simulink model "ZVR_Finale"  (R2019b)
settings: Solver=ode23  StartTime=0.0  StopTime=1  MaxStep=1e-5  RelTol=1e-3
libraries: powerlib x23, powerlib_meascontrol x14, dsparch4 x9, simulink x2
settings Model: Creator=ASUS  LastModifiedBy=ASUS
settings SolverCC: ZeroCrossAlgorithm=Adaptive
settings DebuggingCC: IgnoredZcDiagnostic=none

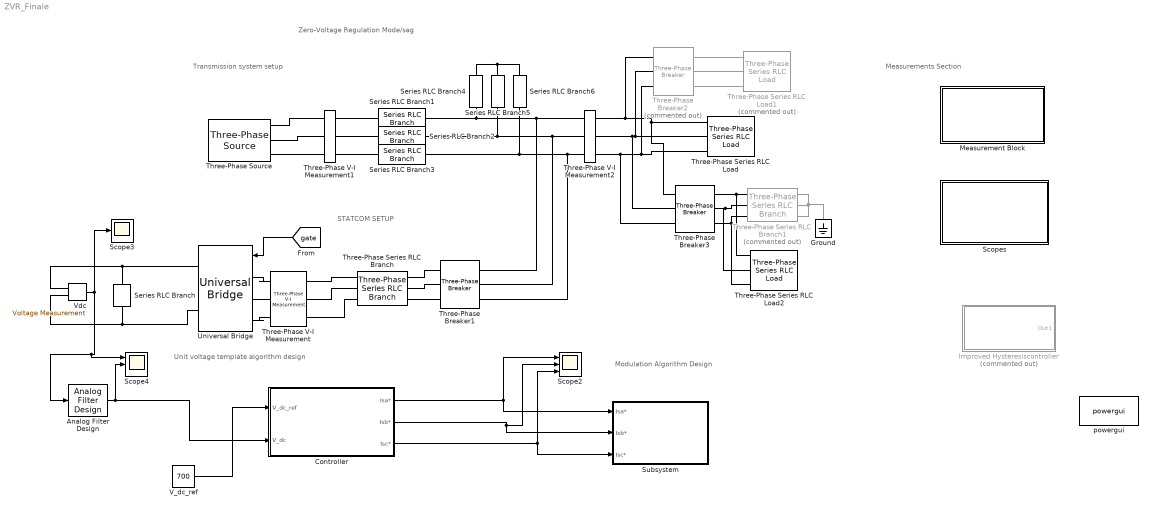
== system ZVR_Finale ==
  note: Zero-Voltage Regulation Mode/sag
  note: Modulation Algorithm Design
  note: Measurements Section
  note: Transmission system setup
  note: Unit voltage template algorithm design
  note: STATCOM SETUP
  Analog Filter Design : dsparch4/Analog Filter Design  method=Butterworth  filttype=Lowpass  N=2  Wlo=100*pi  Whi=80  Rp=2  Rs=40
  Controller : Subsystem
  Ground : powerlib/Elements/Ground  LConnTagsString=a
      settings: SourceProductName=Simscape Electrical
  Improved Hysteresiscontroller : Subsystem  Commented=on
  Measurement Block : Subsystem
  Scope2 : Scope  NumInputPorts=3
  Scope3 : Scope
  Scope4 : Scope  NumInputPorts=3
  Scopes : Subsystem
  Series RLC Branch : powerlib/Elements/Series RLC Branch  LConnTagsString=__new0  RConnTagsString=__new0  BranchType=C  Resistance=1  Inductance=1e-3  SetiL0=off  InitialCurrent=0  Capacitance=10000e-6  Setx0=on  InitialVoltage=700  Measurements=None
      settings: SourceProductName=Simscape Electrical
  Series RLC Branch1 : powerlib/Elements/Series RLC Branch  LConnTagsString=__new0  RConnTagsString=__new0  BranchType=RL  Resistance=0.01  Inductance=1e-3  SetiL0=off  InitialCurrent=0  Capacitance=1e-6  Setx0=off  InitialVoltage=0  Measurements=None
      settings: SourceProductName=Simscape Electrical
  Series RLC Branch2 : powerlib/Elements/Series RLC Branch  LConnTagsString=__new0  RConnTagsString=__new0  BranchType=RL  Resistance=0.01  Inductance=1e-3  SetiL0=off  InitialCurrent=0  Capacitance=1e-6  Setx0=off  InitialVoltage=0  Measurements=None
      settings: SourceProductName=Simscape Electrical
  Series RLC Branch3 : powerlib/Elements/Series RLC Branch  LConnTagsString=__new0  RConnTagsString=__new0  BranchType=RL  Resistance=0.01  Inductance=1e-3  SetiL0=off  InitialCurrent=0  Capacitance=1e-6  Setx0=off  InitialVoltage=0  Measurements=None
      settings: SourceProductName=Simscape Electrical
  Series RLC Branch4 : powerlib/Elements/Series RLC Branch  LConnTagsString=__new0  RConnTagsString=__new0  BranchType=RC  Resistance=5  Inductance=1e-3  SetiL0=off  InitialCurrent=0  Capacitance=5e-6  Setx0=off  InitialVoltage=0  Measurements=None
      settings: SourceProductName=Simscape Electrical
  Series RLC Branch5 : powerlib/Elements/Series RLC Branch  LConnTagsString=__new0  RConnTagsString=__new0  BranchType=RC  Resistance=5  Inductance=1e-3  SetiL0=off  InitialCurrent=0  Capacitance=5e-6  Setx0=off  InitialVoltage=0  Measurements=None
      settings: SourceProductName=Simscape Electrical
  Series RLC Branch6 : powerlib/Elements/Series RLC Branch  LConnTagsString=__new0  RConnTagsString=__new0  BranchType=RC  Resistance=5  Inductance=1e-3  SetiL0=off  InitialCurrent=0  Capacitance=5e-6  Setx0=off  InitialVoltage=0  Measurements=None
      settings: SourceProductName=Simscape Electrical
  Subsystem : Subsystem
  Three-Phase Series RLC Branch : powerlib/Elements/Three-Phase Series RLC Branch  LConnTagsString=A|B|C  RConnTagsString=A|B|C  BranchType=RL  Resistance=0.1  Inductance=4e-3  Capacitance=0  Measurements=None
      settings: SourceProductName=Simscape Electrical
  Three-Phase Series RLC Branch1 : powerlib/Elements/Three-Phase Series RLC Branch  Commented=on  LConnTagsString=A|B|C  RConnTagsString=A|B|C  BranchType=RL  Resistance=0.01  Inductance=10e-3  Capacitance=1e-6  Measurements=None
      settings: SourceProductName=Simscape Electrical
  Three-Phase Series RLC Load : powerlib/Elements/Three-Phase Series RLC Load  LConnTagsString=A|B|C  Configuration=Y (grounded)  NominalVoltage=415  Vabc=[1e3 1e3 1e3]  Vabcp=[1e3 1e3 1e3]  NominalFrequency=50  UnbalancedPower=off  ActivePower=3000  InductivePower=7000  CapacitivePower=0  Pabc=[10e3 9e3 11e3]  QLabc=[100 90 110]  QCabc=[100 90 110]  Pabcp=[10e3 9e3 11e3]  QLabcp=[100 90 110]  QCabcp=[100 90 110]  Measurements=None  LoadType=constant Z
      settings: SourceProductName=Simscape Electrical
  Three-Phase Series RLC Load1 : powerlib/Elements/Three-Phase Series RLC Load  Commented=on  LConnTagsString=A|B|C  Configuration=Y (grounded)  NominalVoltage=415  Vabc=[1e3 1e3 1e3]  Vabcp=[1e3 1e3 1e3]  NominalFrequency=50  UnbalancedPower=off  ActivePower=10e4  InductivePower=3000  CapacitivePower=0  Pabc=[10e3 9e3 11e3]  QLabc=[100 90 110]  QCabc=[100 90 110]  Pabcp=[10e3 9e3 11e3]  QLabcp=[100 90 110]  QCabcp=[100 90 110]  Measurements=None  LoadType=constant Z
      settings: SourceProductName=Simscape Electrical
  Three-Phase Series RLC Load2 : powerlib/Elements/Three-Phase Series RLC Load  LConnTagsString=A|B|C  Configuration=Y (grounded)  NominalVoltage=415  Vabc=[1e3 1e3 1e3]  Vabcp=[1e3 1e3 1e3]  NominalFrequency=50  UnbalancedPower=off  ActivePower=200  InductivePower=10000  CapacitivePower=0  Pabc=[10e3 9e3 11e3]  QLabc=[100 90 110]  QCabc=[100 90 110]  Pabcp=[10e3 9e3 11e3]  QLabcp=[100 90 110]  QCabcp=[100 90 110]  Measurements=None  LoadType=constant Z
      settings: SourceProductName=Simscape Electrical
  Three-Phase V-I Measurement : powerlib/Measurements/Three-Phase V-I Measurement  VoltageMeasurement=phase-to-ground  SetLabelV=on  LabelV=V_stat  Vpu=off  VpuLL=off  CurrentMeasurement=yes  SetLabelI=on  LabelI=I_stat  Ipu=off  Pbase=100e6  Vbase=500e3  OutputType=Complex  PhasorSimulation=off  PSBequivalent=0
      settings: SourceProductName=Simscape Electrical
  Three-Phase V-I Measurement1 : powerlib/Measurements/Three-Phase V-I Measurement  VoltageMeasurement=phase-to-ground  SetLabelV=on  LabelV=Vs  Vpu=off  VpuLL=off  CurrentMeasurement=yes  SetLabelI=on  LabelI=Is  Ipu=off  Pbase=100e6  Vbase=500e3  OutputType=Complex  PhasorSimulation=off  PSBequivalent=0
      settings: SourceProductName=Simscape Electrical
  Three-Phase V-I Measurement2 : powerlib/Measurements/Three-Phase V-I Measurement  VoltageMeasurement=phase-to-ground  SetLabelV=on  LabelV=Vr  Vpu=off  VpuLL=off  CurrentMeasurement=yes  SetLabelI=on  LabelI=Ir  Ipu=off  Pbase=100e6  Vbase=500e3  OutputType=Complex  PhasorSimulation=off  PSBequivalent=0
      settings: SourceProductName=Simscape Electrical
  Three-Phase Breaker1 : powerlib/Elements/Three-Phase Breaker  InitialState=open  SwitchA=on  SwitchB=on  SwitchC=on  SwitchTimes=[0.2 0.6]  External=off  BreakerResistance=0.01  SnubberResistance=1e6  SnubberCapacitance=inf  Measurements=None
      settings: SourceProductName=Simscape Electrical
  Three-Phase Breaker2 : powerlib/Elements/Three-Phase Breaker  Commented=on  InitialState=open  SwitchA=on  SwitchB=on  SwitchC=on  SwitchTimes=[0.1 0.5]  External=off  BreakerResistance=0.01  SnubberResistance=1e6  SnubberCapacitance=inf  Measurements=None
      settings: SourceProductName=Simscape Electrical
  Three-Phase Breaker3 : powerlib/Elements/Three-Phase Breaker  InitialState=open  SwitchA=on  SwitchB=on  SwitchC=on  SwitchTimes=[0.1 0.6]  External=off  BreakerResistance=0.01  SnubberResistance=1e6  SnubberCapacitance=inf  Measurements=None
      settings: SourceProductName=Simscape Electrical
  Three-Phase Source : powerlib/Electrical Sources/Three-Phase Source  InternalConnection=Yg  VoltagePhases=off  Voltage=415  PhaseAngle=0  Voltage_phases=[25e3 25e3 25e3]/sqrt(3)  PhaseAngles_phases=[0 -120 +120]  Frequency=50  NonIdealSource=on  SpecifyImpedance=off  Resistance=0.04  Inductance=0.5e-3  ShortCircuitLevel=100e6  BaseVoltage=415  XRratio=7  BusType=swing  Pref=10e3  Qref=0  Prefabc=[10e3, 10e3, 10e3]  Qrefabc=[0, 0, 0]  Qmin=-inf  Qmax=inf
      settings: SourceProductName=Simscape Electrical
  Universal Bridge : powerlib/Power Electronics/Universal Bridge  Arms=3  SnubberResistance=1e5  SnubberCapacitance=inf  Device=IGBT / Diodes  Ron=1e-3  Lon=0  ForwardVoltages="[  0  0  ]"  ForwardVoltage=0  GTOparameters=[ 10e-6 , 20e-6 ]  IGBTparameters=[ 1e-6 , 2e-6 ]  Measurements=None  Measurements_2=None  converterType=Rectifier
      settings: SourceProductName=Simscape Electrical
  V_dc_ref : Constant  Value=700
  Vdc : powerlib/Measurements/Voltage Measurement  PhasorSimulation=off  OutputType=Complex  PSBequivalent=0
      settings: SourceProductName=Simscape Electrical
  powergui : powerlib/powergui  Priority=1  SimulationMode=Discrete  SampleTime=1e-6  frequency=60  Iterations=50  frequencyindice=0  Pbase=100e6  ErrMax=1e-4  UnitsV=kV  UnitsW=MW  buscounter=0  FunctionMessages=off  echomessages=off  EnableUseOfTLC=off  CurrentSourceSwitches=off  DisableSnubberDevices=off  DisableRonSwitches=off  DisableVfSwitches=off  DisplayEquations=off  AutomaticDiscreteSolvers=off  SolverType=Tustin/Backward Euler (TBE)  Interpol=off  ExternalGateDelay=off  methode=off  Ts=100  x0status=blocks  SPID=on  SwTol=0  HookPort=off  NonlinearTolerance=1e-4  nMaxIteration=100  ContinueOnMaxIteration=off  RestoreLinks=warning  ResistiveCurrentMeasurement=off  Frange=[0:2:500]  Ylog=off  Xlog=on  ShowGrid=off  save=off  variable=ZData  structure=0  ZoomFFT=off  StartTime=0.0  cycles=1  DisplayStyle=1  fundamental=60  FreqAxis=off  MaxFrequency=1000  frequencyindicesteady=1  RmsSteady=1  display=off
      settings: SourceProductName=Simscape Electrical
  wires:
  V_dc_ref/1 -> Controller/1(V_dc_ref)
  Controller/1(Isa*) -> Subsystem/1(Isa*), Scope2/1
  Controller/2(Isb*) -> Subsystem/2(Isb*), Scope2/2
  Controller/3(Isc*) -> Subsystem/3(Isc*), Scope2/3
  Vdc/1 -> Scope4/1, Analog Filter Design/1, Scope3/1
  Analog Filter Design/1 -> Scope4/2, Controller/2(V_dc)
  [gate] -> Universal Bridge/1
  connections:
  Three-Phase Source/RConn1 -- Three-Phase V-I Measurement1/LConn1
  Three-Phase Source/RConn2 -- Three-Phase V-I Measurement1/LConn2
  Three-Phase Source/RConn3 -- Three-Phase V-I Measurement1/LConn3
  Series RLC Branch5/LConn1 -- Series RLC Branch2/RConn1 -- Three-Phase Breaker1/RConn2 -- Three-Phase V-I Measurement2/LConn2
  Series RLC Branch6/LConn1 -- Series RLC Branch3/RConn1 -- Three-Phase Breaker1/RConn3 -- Three-Phase V-I Measurement2/LConn3
  Three-Phase Series RLC Load/LConn1 -- Three-Phase Breaker2/LConn1 -- Three-Phase V-I Measurement2/RConn1 -- Three-Phase Breaker3/LConn1
  Three-Phase Series RLC Load/LConn2 -- Three-Phase Breaker3/LConn2 -- Three-Phase V-I Measurement2/RConn2 -- Three-Phase Breaker2/LConn2
  Three-Phase V-I Measurement2/RConn3 -- Three-Phase Breaker3/LConn3 -- Three-Phase Breaker2/LConn3 -- Three-Phase Series RLC Load/LConn3
  Series RLC Branch4/LConn1 -- Series RLC Branch1/RConn1 -- Three-Phase Breaker1/RConn1 -- Three-Phase V-I Measurement2/LConn1
  Series RLC Branch4/RConn1 -- Series RLC Branch6/RConn1 -- Series RLC Branch5/RConn1
  Series RLC Branch/LConn1 -- Vdc/LConn1 -- Universal Bridge/RConn1
  Series RLC Branch/RConn1 -- Universal Bridge/RConn2 -- Vdc/LConn2
  Three-Phase Series RLC Branch/RConn3 -- Three-Phase Breaker1/LConn3
  Three-Phase Series RLC Branch/RConn1 -- Three-Phase Breaker1/LConn1
  Three-Phase Series RLC Branch/RConn2 -- Three-Phase Breaker1/LConn2
  Three-Phase V-I Measurement/LConn1 -- Universal Bridge/LConn1
  Universal Bridge/LConn2 -- Three-Phase V-I Measurement/LConn2
  Universal Bridge/LConn3 -- Three-Phase V-I Measurement/LConn3
  Three-Phase V-I Measurement/RConn1 -- Three-Phase Series RLC Branch/LConn1
  Three-Phase V-I Measurement/RConn2 -- Three-Phase Series RLC Branch/LConn2
  Three-Phase V-I Measurement/RConn3 -- Three-Phase Series RLC Branch/LConn3
  Series RLC Branch1/LConn1 -- Three-Phase V-I Measurement1/RConn1
  Series RLC Branch2/LConn1 -- Three-Phase V-I Measurement1/RConn2
  Series RLC Branch3/LConn1 -- Three-Phase V-I Measurement1/RConn3
  Three-Phase Breaker2/RConn1 -- Three-Phase Series RLC Load1/LConn1
  Three-Phase Breaker2/RConn2 -- Three-Phase Series RLC Load1/LConn2
  Three-Phase Breaker2/RConn3 -- Three-Phase Series RLC Load1/LConn3
  Three-Phase Series RLC Branch1/RConn1 -- Ground/LConn1 -- Three-Phase Series RLC Branch1/RConn2 -- Three-Phase Series RLC Branch1/RConn3
  Three-Phase Breaker3/RConn1 -- Three-Phase Series RLC Load2/LConn1 -- Three-Phase Series RLC Branch1/LConn1
  Three-Phase Breaker3/RConn2 -- Three-Phase Series RLC Branch1/LConn2 -- Three-Phase Series RLC Load2/LConn2
  Three-Phase Breaker3/RConn3 -- Three-Phase Series RLC Load2/LConn3 -- Three-Phase Series RLC Branch1/LConn3

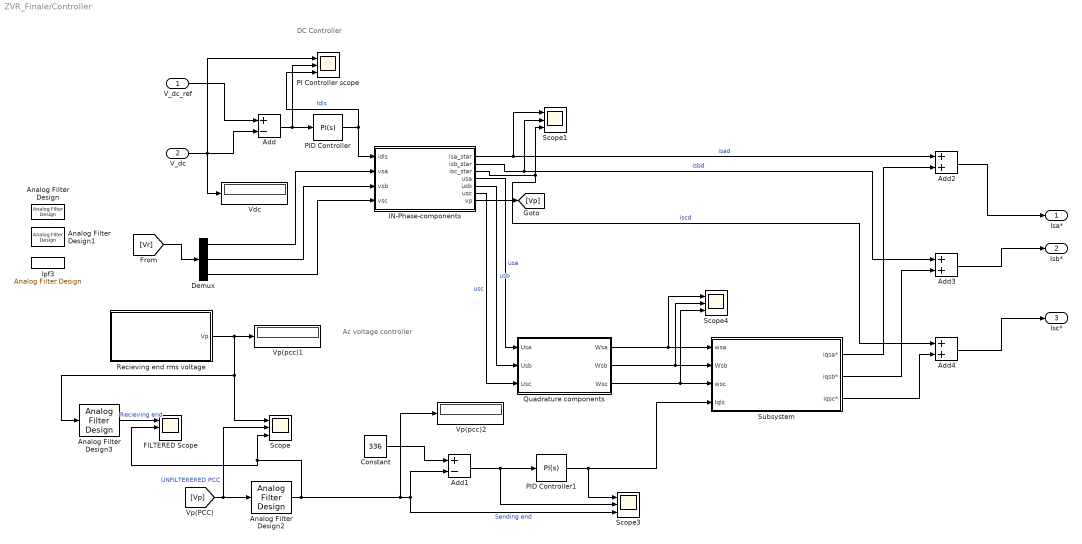
== system ZVR_Finale/Controller ==
  note: Ac voltage controller
  note: DC Controller
  V_dc_ref : Inport
  V_dc : Inport  Port=2
  Add : Sum  Inputs=+-
  Add1 : Sum  Inputs=+-
  Add2 : Sum
  Add3 : Sum
  Add4 : Sum
  Analog Filter Design : dsparch4/Analog Filter Design  method=Butterworth  filttype=Lowpass  N=2  Wlo=20000*2*pi  Whi=80  Rp=2  Rs=40
  Analog Filter Design1 : dsparch4/Analog Filter Design  method=Butterworth  filttype=Lowpass  N=2  Wlo=20000*2*pi  Whi=80  Rp=2  Rs=40
  Analog Filter Design2 : dsparch4/Analog Filter Design  method=Butterworth  filttype=Lowpass  N=2  Wlo=50*pi  Whi=80  Rp=2  Rs=40
  Analog Filter Design3 : dsparch4/Analog Filter Design  method=Butterworth  filttype=Lowpass  N=2  Wlo=50*pi  Whi=80  Rp=2  Rs=40
  Constant : Constant  Value=336
  Demux : Demux  Outputs=3
  FILTERED Scope : Scope  NumInputPorts=3
  IN-Phase-components : MATLAB Function  TreatAsAtomicUnit=on
  PI Controller scope : Scope  NumInputPorts=3
  PID Controller : simulink/Continuous/PID Controller  Controller=PI  Form=Parallel  TimeDomain=Continuous-time  SampleTime=-1  IntegratorMethod=Forward Euler  FilterMethod=Forward Euler  ControllerParametersSource=internal  P=3  I=8  D=0  UseFilter=on  N=100  TunerSelectOption=Transfer Function Based (PID Tuner App)  InitialConditionSource=internal  InitialConditionForIntegrator=0  InitialConditionForFilter=0  DifferentiatorICPrevScaledInput=0  ExternalReset=none  TrackingMode=off  Kt=1  LimitOutput=off  UpperSaturationLimit=inf  LowerSaturationLimit=-inf  LinearizeAsGain=on  AntiWindupMode=none  Kb=1  POutMin=[]  POutMax=[]  IOutMin=[]  IOutMax=[]  DOutMin=[]  DOutMax=[]  NOutMin=[]  NOutMax=[]  SumOutMin=[]  SumOutMax=[]  SaturationOutMin=[]  SaturationOutMax=[]  PParamMin=[]  PParamMax=[]  IParamMin=[]  IParamMax=[]  DParamMin=[]  DParamMax=[]  NParamMin=[]  NParamMax=[]  KbParamMin=[]  KbParamMax=[]  KtParamMin=[]  KtParamMax=[]  KbOutMin=[]  KbOutMax=[]  KtOutMin=[]  KtOutMax=[]  IntegratorOutMin=[]  IntegratorOutMax=[]  FilterOutMin=[]  FilterOutMax=[]  SumI1OutMin=[]  SumI1OutMax=[]  SumI2OutMin=[]  SumI2OutMax=[]  SumI3OutMin=[]  SumI3OutMax=[]  SumI4OutMin=[]  SumI4OutMax=[]  SumDOutMin=[]  SumDOutMax=[]  DifferentiatorOutMin=[]  DifferentiatorOutMax=[]  FilterDiffOutCoefMin=[]  FilterDiffOutCoefMax=[]  ReciprocalOutMin=[]  ReciprocalOutMax=[]  SumDenOutMin=[]  SumDenOutMax=[]  SumNumOutMin=[]  SumNumOutMax=[]  DivideOutMin=[]  DivideOutMax=[]  IntegratorContinuousStateAttributes=''  IntegratorStateMustResolveToSignalObject=off  IntegratorRTWStateStorageClass=Auto  FilterContinuousStateAttributes=''  FilterStateMustResolveToSignalObject=off  FilterRTWStateStorageClass=Auto  ParallelPVariant=InternalParameters  IdealPVariant=Disabled  IVariant=InternalParameters  DVariant=Disabled  IntegratorVariant=Continuous  SatVariant=Disabled  AWVariant=Passthrough  PCopyVariant=Disabled  TRVariant=Disabled  FdbkBlocksVariant=Forward  IdealPFdbkVariant=Disabled  SatFdbkVariant=Disabled  DerivativeFilterVariant=Disabled  NVariant=Disabled  NCopyVariant=Disabled_SignalSpec  FilterICVariant=Disabled  IntegratorICVariant=InternalICs  ExternalResetVariant=Disabled  TRSumVariant=Passthrough  SumFdbkVariant=Disabled  SumVariant=Sum_PI
  PID Controller1 : simulink/Continuous/PID Controller  Controller=PI  Form=Parallel  TimeDomain=Continuous-time  SampleTime=-1  IntegratorMethod=Forward Euler  FilterMethod=Forward Euler  ControllerParametersSource=internal  P=1.2  I=0.6  D=0  UseFilter=on  N=100  TunerSelectOption=Transfer Function Based (PID Tuner App)  InitialConditionSource=internal  InitialConditionForIntegrator=0  InitialConditionForFilter=0  DifferentiatorICPrevScaledInput=0  ExternalReset=none  TrackingMode=off  Kt=1  LimitOutput=off  UpperSaturationLimit=inf  LowerSaturationLimit=-inf  LinearizeAsGain=on  AntiWindupMode=none  Kb=1  POutMin=[]  POutMax=[]  IOutMin=[]  IOutMax=[]  DOutMin=[]  DOutMax=[]  NOutMin=[]  NOutMax=[]  SumOutMin=[]  SumOutMax=[]  SaturationOutMin=[]  SaturationOutMax=[]  PParamMin=[]  PParamMax=[]  IParamMin=[]  IParamMax=[]  DParamMin=[]  DParamMax=[]  NParamMin=[]  NParamMax=[]  KbParamMin=[]  KbParamMax=[]  KtParamMin=[]  KtParamMax=[]  KbOutMin=[]  KbOutMax=[]  KtOutMin=[]  KtOutMax=[]  IntegratorOutMin=[]  IntegratorOutMax=[]  FilterOutMin=[]  FilterOutMax=[]  SumI1OutMin=[]  SumI1OutMax=[]  SumI2OutMin=[]  SumI2OutMax=[]  SumI3OutMin=[]  SumI3OutMax=[]  SumI4OutMin=[]  SumI4OutMax=[]  SumDOutMin=[]  SumDOutMax=[]  DifferentiatorOutMin=[]  DifferentiatorOutMax=[]  FilterDiffOutCoefMin=[]  FilterDiffOutCoefMax=[]  ReciprocalOutMin=[]  ReciprocalOutMax=[]  SumDenOutMin=[]  SumDenOutMax=[]  SumNumOutMin=[]  SumNumOutMax=[]  DivideOutMin=[]  DivideOutMax=[]  IntegratorContinuousStateAttributes=''  IntegratorStateMustResolveToSignalObject=off  IntegratorRTWStateStorageClass=Auto  FilterContinuousStateAttributes=''  FilterStateMustResolveToSignalObject=off  FilterRTWStateStorageClass=Auto  ParallelPVariant=InternalParameters  IdealPVariant=Disabled  IVariant=InternalParameters  DVariant=Disabled  IntegratorVariant=Continuous  SatVariant=Disabled  AWVariant=Passthrough  PCopyVariant=Disabled  TRVariant=Disabled  FdbkBlocksVariant=Forward  IdealPFdbkVariant=Disabled  SatFdbkVariant=Disabled  DerivativeFilterVariant=Disabled  NVariant=Disabled  NCopyVariant=Disabled_SignalSpec  FilterICVariant=Disabled  IntegratorICVariant=InternalICs  ExternalResetVariant=Disabled  TRSumVariant=Passthrough  SumFdbkVariant=Disabled  SumVariant=Sum_PI
  "Quadrature components " : Subsystem
  Recieving end rms voltage : Subsystem
  Scope{,1,3..4} (4 alike) : Scope  NumInputPorts=3
  Subsystem : Subsystem
  Vdc : Display
  Vp(pcc)1 : Display
  Vp(pcc)2 : Display
  lpf3 : dsparch4/Analog Filter Design  method=Butterworth  filttype=Lowpass  N=2  Wlo=20000*2*pi  Whi=80  Rp=2  Rs=40
  Isa* : Outport
  Isb* : Outport  Port=2
  Isc* : Outport  Port=3
  wires:
  V_dc_ref/1 -> Add/1
  V_dc/1 -> PI Controller scope/1, Add/2, Vdc/1
  Add/1 -> PI Controller scope/2, PID Controller/1
  PID Controller/1 -> PI Controller scope/3, IN-Phase-components/1(idls)  "Idls"
  [Vr] -> Demux/1
  IN-Phase-components/1(isa_star) -> Add2/1, Scope1/1  "isad"
  IN-Phase-components/2(isb_star) -> Add3/1, Scope1/2  "isbd"
  IN-Phase-components/3(isc_star) -> Add4/1, Scope1/3  "iscd"
  IN-Phase-components/4(usa) -> "Quadrature components "/1(Usa)  "usa"
  IN-Phase-components/5(usb) -> "Quadrature components "/2(Usb)  "usb"
  IN-Phase-components/6(usc) -> "Quadrature components "/3(Usc)  "usc"
  Demux/1 -> IN-Phase-components/2(vsa)
  Demux/2 -> IN-Phase-components/3(vsb)
  Demux/3 -> IN-Phase-components/4(vsc)
  "Quadrature components "/1(Wsa) -> Scope4/1, Subsystem/1(wsa)
  Recieving end rms voltage/1(Vp) -> Analog Filter Design3/1, Scope/1, Vp(pcc)1/1
  IN-Phase-components/7(vp) -> [Vp]
  Constant/1 -> Add1/1
  Analog Filter Design2/1 -> Scope/3, FILTERED Scope/2, Vp(pcc)2/1, Add1/2, Scope3/3  "Sending end"
  Add1/1 -> Scope3/2, PID Controller1/1
  PID Controller1/1 -> Scope3/1, Subsystem/4(Iqls)
  "Quadrature components "/2(Wsb) -> Scope4/2, Subsystem/2(Wsb)
  "Quadrature components "/3(Wsc) -> Scope4/3, Subsystem/3(wsc)
  Subsystem/1(iqsa*) -> Add2/2
  Add2/1 -> Isa*/1
  Subsystem/2(iqsb*) -> Add3/2
  Subsystem/3(iqsc*) -> Add4/2
  Add3/1 -> Isb*/1
  Add4/1 -> Isc*/1
  [Vp] -> Scope/2, Analog Filter Design2/1  "UNFILTERERED PCC"
  Analog Filter Design3/1 -> FILTERED Scope/1  "Recieving end"

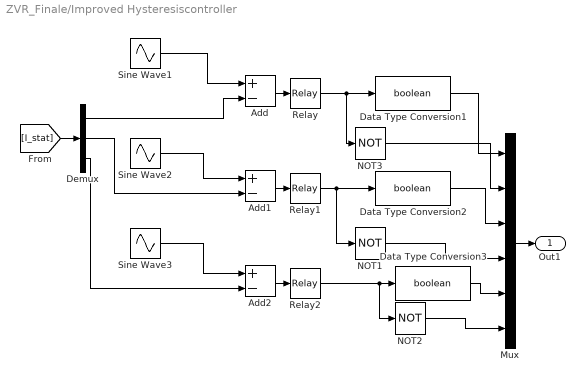
== system ZVR_Finale/Improved Hysteresiscontroller ==
  Add : Sum  Inputs=+-
  Add1 : Sum  Inputs=+-
  Add2 : Sum  Inputs=+-
  Data Type Conversion1 : DataTypeConversion  OutDataTypeStr=boolean
  Data Type Conversion2 : DataTypeConversion  OutDataTypeStr=boolean
  Data Type Conversion3 : DataTypeConversion  OutDataTypeStr=boolean
  Demux : Demux  Outputs=3
  Mux : Mux  Inputs=6
  NOT1 : Logic  Operator=NOT  IconShape=distinctive  AllPortsSameDT=off  OutDataTypeStr=boolean
  NOT2 : Logic  Operator=NOT  IconShape=distinctive  AllPortsSameDT=off  OutDataTypeStr=boolean
  NOT3 : Logic  Operator=NOT  IconShape=distinctive  AllPortsSameDT=off  OutDataTypeStr=boolean
  Relay : Relay  OnSwitchValue=0.1  OffSwitchValue=-0.1
  Relay1 : Relay  OnSwitchValue=0.1  OffSwitchValue=-0.1
  Relay2 : Relay  OnSwitchValue=0.1  OffSwitchValue=-0.1
  Sine Wave1 : Sin  Amplitude=5  Frequency=100*pi  SampleTime=0
  Sine Wave2 : Sin  Amplitude=5  Frequency=100*pi  Phase=-2*pi/3  SampleTime=0
  Sine Wave3 : Sin  Amplitude=5  Frequency=100*pi  Phase=2*pi/3  SampleTime=0
  Out1 : Outport
  wires:
  Data Type Conversion3/1 -> Mux/5
  Relay/1 -> NOT3/1, Data Type Conversion1/1
  Sine Wave1/1 -> Add/1
  Add2/1 -> Relay2/1
  Sine Wave2/1 -> Add1/1
  Relay1/1 -> NOT1/1, Data Type Conversion2/1
  Sine Wave3/1 -> Add2/1
  Data Type Conversion1/1 -> Mux/1
  NOT1/1 -> Mux/4
  NOT3/1 -> Mux/2
  Add1/1 -> Relay1/1
  Relay2/1 -> Data Type Conversion3/1, NOT2/1
  [I_stat] -> Demux/1
  Demux/2 -> Add1/2
  Add/1 -> Relay/1
  Demux/1 -> Add/2
  NOT2/1 -> Mux/6
  Data Type Conversion2/1 -> Mux/3
  Demux/3 -> Add2/2
  Mux/1 -> Out1/1

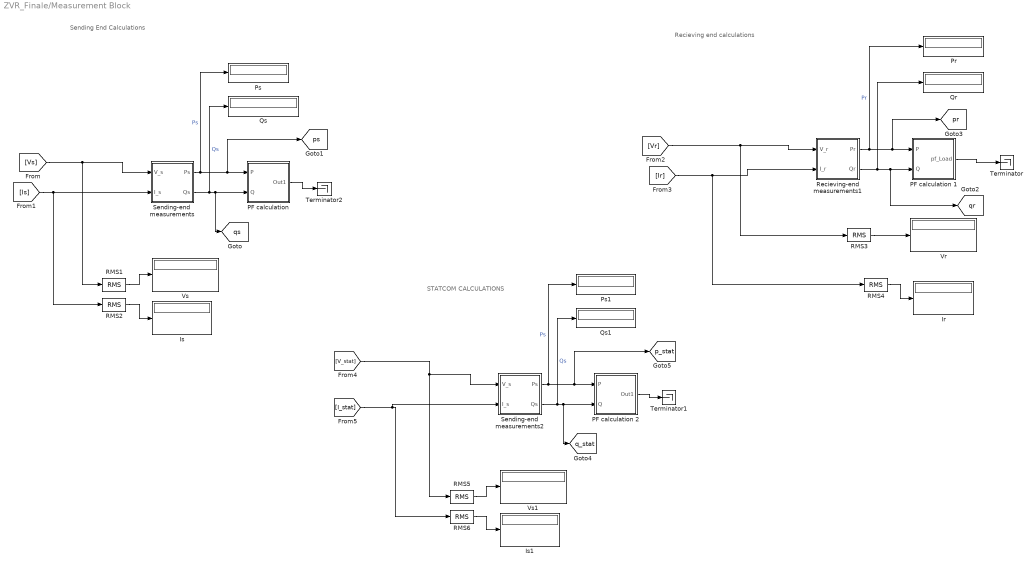
== system ZVR_Finale/Measurement Block ==
  note: STATCOM CALCULATIONS
  note: Recieving end calculations
  note: Sending End Calculations
  Ir : Display
  Is : Display
  Is1 : Display
  "PF calculation " : Subsystem
  PF calculation 1 : Subsystem
  PF calculation 2 : Subsystem
  Pr : Display
  Ps : Display
  Ps1 : Display
  Qr : Display
  Qs : Display
      settings: Format=short_e
  Qs1 : Display
  RMS{1..6} (6 alike) : powerlib_meascontrol/Measurements/RMS  TrueRMS=on  Freq=60  RMSInit=120  Ts=0
      settings: SourceProductName=Simscape Electrical
  Recieving-end measurements1 : Subsystem
  Sending-end measurements : Subsystem
  Sending-end measurements2 : Subsystem
  Terminator : Terminator
  Terminator1 : Terminator
  Terminator2 : Terminator
  Vr : Display
  Vs : Display
  Vs1 : Display
  tag scope: p_stat=global, pr=global, ps=global, q_stat=global, qr=global, qs=global
  wires:
  Sending-end measurements/1(Ps) -> Ps/1, [ps], "PF calculation "/1(P)  "Ps"
  Sending-end measurements/2(Qs) -> Qs/1, [qs], "PF calculation "/2(Q)  "Qs"
  [Is] -> RMS2/1, Sending-end measurements/2(I_s)
  Recieving-end measurements1/2(Qr) -> Qr/1, [qr], PF calculation 1/2(Q)
  Recieving-end measurements1/1(Pr) -> Pr/1, [pr], PF calculation 1/1(P)  "Pr"
  RMS1/1 -> Vs/1
  RMS2/1 -> Is/1
  [Vs] -> Sending-end measurements/1(V_s), RMS1/1
  RMS3/1 -> Vr/1
  [Vr] -> RMS3/1, Recieving-end measurements1/1(V_r)
  RMS4/1 -> Ir/1
  [Ir] -> RMS4/1, Recieving-end measurements1/2(I_r)
  Sending-end measurements2/2(Qs) -> Qs1/1, [q_stat], PF calculation 2/2(Q)  "Qs"
  Sending-end measurements2/1(Ps) -> Ps1/1, [p_stat], PF calculation 2/1(P)  "Ps"
  [V_stat] -> Sending-end measurements2/1(V_s), RMS5/1
  RMS5/1 -> Vs1/1
  RMS6/1 -> Is1/1
  [I_stat] -> Sending-end measurements2/2(I_s), RMS6/1
  PF calculation 1/1(pf_Load) -> Terminator/1
  PF calculation 2/1(Out1) -> Terminator1/1
  "PF calculation "/1(Out1) -> Terminator2/1

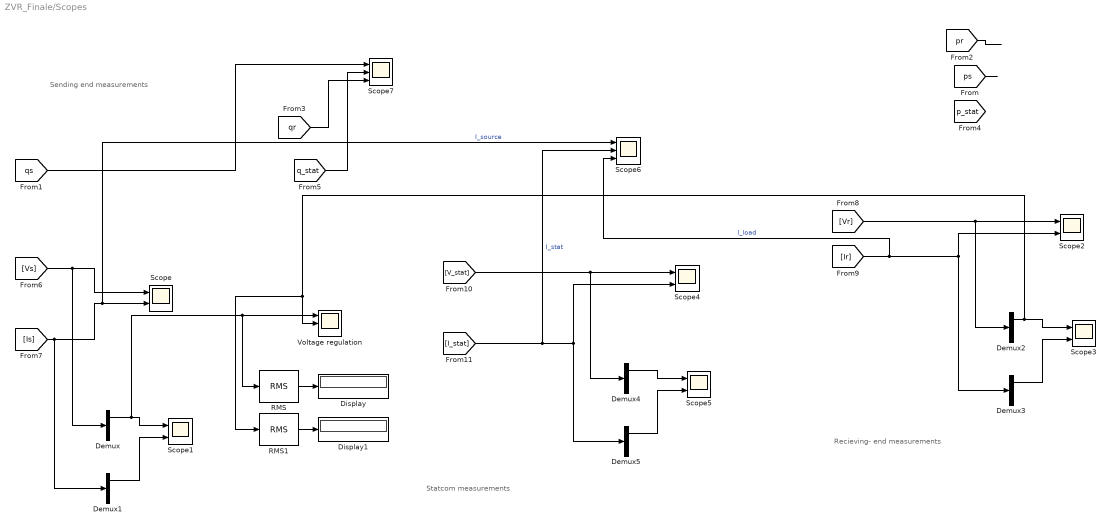
== system ZVR_Finale/Scopes ==
  note: Recieving- end measurements
  note: Statcom measurements
  note: Sending end measurements
  Demux{,1..5} (6 alike) : Demux  Outputs=3
  Display : Display
  Display1 : Display
  RMS : powerlib_meascontrol/Measurements/RMS  TrueRMS=on  Freq=60  RMSInit=120  Ts=0
      settings: SourceProductName=Simscape Electrical
  RMS1 : powerlib_meascontrol/Measurements/RMS  TrueRMS=on  Freq=60  RMSInit=120  Ts=0
      settings: SourceProductName=Simscape Electrical
  Scope{,1..5} (6 alike) : Scope  NumInputPorts=2
  Scope6 : Scope  NumInputPorts=3
  Scope7 : Scope  NumInputPorts=3
  Voltage regulation : Scope  NumInputPorts=3
  wires:
  [ps] -> ?
  [qr] -> Scope7/3
  [pr] -> ?
  [qs] -> Scope7/1
  [Vs] -> Demux/1, Scope/1
  [Is] -> Demux1/1, Scope6/1, Scope/2  "I_source"
  Demux/1 -> RMS/1, Voltage regulation/1, Scope1/1
  Demux1/1 -> Scope1/2
  Demux3/1 -> Scope3/2
  Demux2/1 -> RMS1/1, Voltage regulation/2, Scope3/1
  [Ir] -> Scope6/3, Demux3/1, Scope2/2  "I_load"
  [Vr] -> Demux2/1, Scope2/1
  [V_stat] -> Scope4/1, Demux4/1
  [I_stat] -> Scope6/2, Scope4/2, Demux5/1  "I_stat"
  Demux4/1 -> Scope5/1
  Demux5/1 -> Scope5/2
  [q_stat] -> Scope7/2
  RMS1/1 -> Display1/1
  RMS/1 -> Display/1

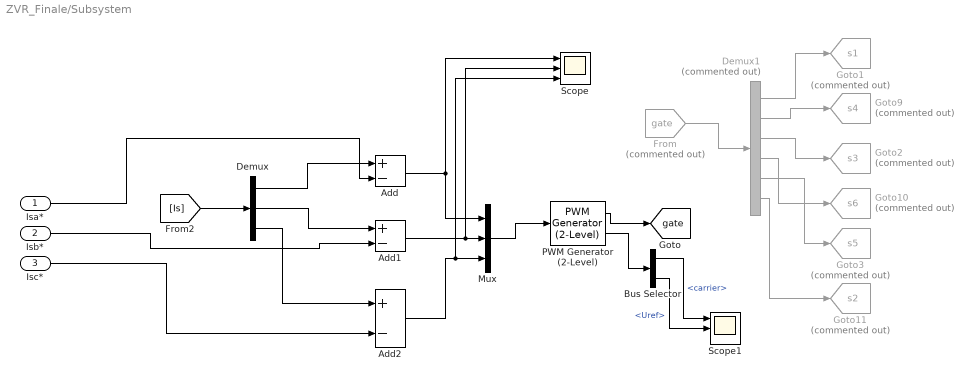
== system ZVR_Finale/Subsystem ==
  Isa* : Inport
  Isb* : Inport  Port=2
  Isc* : Inport  Port=3
  Add : Sum  Inputs=+-
  Add1 : Sum  Inputs=+-
  Add2 : Sum  Inputs=+-
  Bus Selector : BusSelector  OutputSignals=carrier,Uref
  Demux : Demux  Outputs=3
  Demux1 : Demux  Commented=on  Outputs=6
  From : From  Commented=on  GotoTag=gate  TagVisibility=global
  Goto1 : Goto  Commented=on  GotoTag=s1  TagVisibility=global
  Goto10 : Goto  Commented=on  GotoTag=s6  TagVisibility=global
  Goto11 : Goto  Commented=on  GotoTag=s2  TagVisibility=global
  Goto2 : Goto  Commented=on  GotoTag=s3  TagVisibility=global
  Goto3 : Goto  Commented=on  GotoTag=s5  TagVisibility=global
  Goto9 : Goto  Commented=on  GotoTag=s4  TagVisibility=global
  Mux : Mux  Inputs=3
  PWM Generator (2-Level) : powerlib_meascontrol/Pulse & Signal Generators/PWM Generator (2-Level)  ModulatorType=Three-phase bridge (6 pulses)  ModulatorMode=Unsynchronized  Fc=12000  Pc=0  nF=10000  MinMax=[ -500 500]  SamplingTechnique=Symmetrical regular (single edge)  ModulatingSignals=off  m=0.8  Freq=60  Phase=0  Ts=0  ShowCarrierOutport=on
  Scope : Scope  NumInputPorts=3
  Scope1 : Scope  NumInputPorts=3
  tag scope: gate=global
  wires:
  Add/1 -> Scope/1, Mux/1
  Add1/1 -> Scope/2, Mux/2
  Demux/3 -> Add2/1
  PWM Generator (2-Level)/1 -> [gate]
  Add2/1 -> Scope/3, Mux/3
  [Is] -> Demux/1
  Demux/2 -> Add1/1
  Mux/1 -> PWM Generator (2-Level)/1
  Isb*/1 -> Add1/2
  Demux/1 -> Add/1
  Isa*/1 -> Add/2
  Isc*/1 -> Add2/2
  PWM Generator (2-Level)/2 -> Bus Selector/1
  Bus Selector/1 -> Scope1/1  "<carrier>"
  Bus Selector/2 -> Scope1/2  "<Uref>"
  From/1 -> Demux1/1
  Demux1/1 -> Goto1/1
  Demux1/2 -> Goto9/1
  Demux1/3 -> Goto2/1
  Demux1/4 -> Goto10/1
  Demux1/5 -> Goto3/1
  Demux1/6 -> Goto11/1

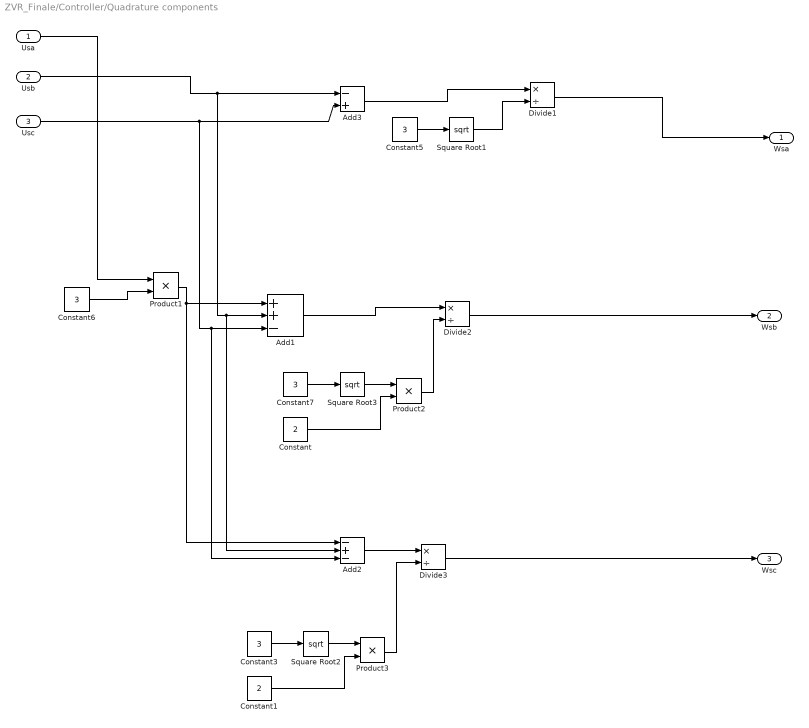
== system ZVR_Finale/Controller/Quadrature components  ==
  Usa : Inport
  Usb : Inport  Port=2
  Usc : Inport  Port=3
  Add1 : Sum  Inputs=++-
  Add2 : Sum  Inputs=-+-
  Add3 : Sum  Inputs=-+
  Constant : Constant  Value=2
  Constant1 : Constant  Value=2
  Constant{3,5..7} (4 alike) : Constant  Value=3
  Divide1 : Product  Inputs=*/
  Divide2 : Product  Inputs=*/
  Divide3 : Product  Inputs=*/
  Product1 : Product
  Product2 : Product
  Product3 : Product
  Square Root1 : Sqrt  SaturateOnIntegerOverflow=on
  Square Root2 : Sqrt  SaturateOnIntegerOverflow=on
  Square Root3 : Sqrt  SaturateOnIntegerOverflow=on
  Wsa : Outport
  Wsb : Outport  Port=2
  Wsc : Outport  Port=3
  wires:
  Divide1/1 -> Wsa/1
  Usb/1 -> Add3/1, Add2/2, Add1/2
  Usc/1 -> Add2/3, Add1/3, Add3/2
  Add3/1 -> Divide1/1
  Constant5/1 -> Square Root1/1
  Square Root1/1 -> Divide1/2
  Constant6/1 -> Product1/2
  Usa/1 -> Product1/1
  Product1/1 -> Add2/1, Add1/1
  Add1/1 -> Divide2/1
  Constant7/1 -> Square Root3/1
  Square Root3/1 -> Product2/1
  Constant/1 -> Product2/2
  Product2/1 -> Divide2/2
  Divide2/1 -> Wsb/1
  Product3/1 -> Divide3/2
  Constant1/1 -> Product3/2
  Square Root2/1 -> Product3/1
  Constant3/1 -> Square Root2/1
  Add2/1 -> Divide3/1
  Divide3/1 -> Wsc/1

== system ZVR_Finale/Controller/Recieving end rms voltage ==
  Analog Filter Design2 : dsparch4/Analog Filter Design  method=Butterworth  filttype=Lowpass  N=2  Wlo=20000*2*pi  Whi=80  Rp=2  Rs=40
  Analog Filter Design3 : dsparch4/Analog Filter Design  method=Butterworth  filttype=Lowpass  N=2  Wlo=20000*2*pi  Whi=80  Rp=2  Rs=40
  Demux1 : Demux  Outputs=3
  Vp(PCC voltage) : Subsystem
  lpf1 : dsparch4/Analog Filter Design  method=Butterworth  filttype=Lowpass  N=2  Wlo=20000*2*pi  Whi=80  Rp=2  Rs=40
  Vp : Outport
  wires:
  Demux1/3 -> lpf1/1
  Demux1/1 -> Analog Filter Design2/1
  Demux1/2 -> Analog Filter Design3/1
  Analog Filter Design2/1 -> Vp(PCC voltage)/1(Vsa)
  lpf1/1 -> Vp(PCC voltage)/3(Vsc)
  [Vs] -> Demux1/1
  Vp(PCC voltage)/1(Vp) -> Vp/1  "Vp"
  Analog Filter Design3/1 -> Vp(PCC voltage)/2(Vsb)

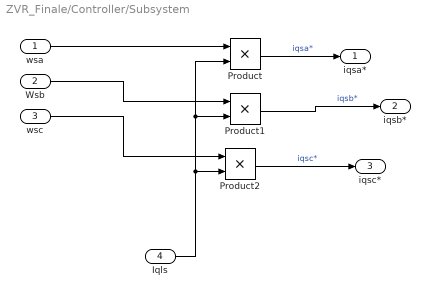
== system ZVR_Finale/Controller/Subsystem ==
  wsa : Inport
  Wsb : Inport  Port=2
  wsc : Inport  Port=3
  Iqls : Inport  Port=4
  Product : Product
  Product1 : Product
  Product2 : Product
  iqsa* : Outport
  iqsb* : Outport  Port=2
  iqsc* : Outport  Port=3
  wires:
  Product1/1 -> iqsb*/1  "iqsb*"
  wsa/1 -> Product/1
  Iqls/1 -> Product2/2, Product1/2, Product/2
  Wsb/1 -> Product1/1
  wsc/1 -> Product2/1
  Product2/1 -> iqsc*/1  "iqsc*"
  Product/1 -> iqsa*/1  "iqsa*"

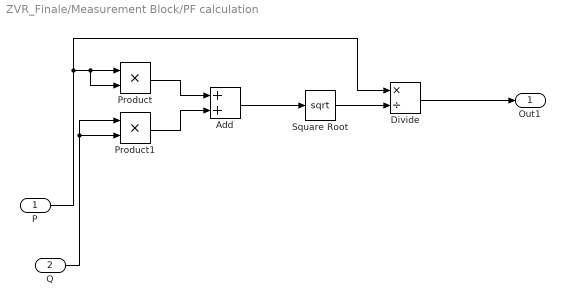
== system ZVR_Finale/Measurement Block/PF calculation  ==
  P : Inport
  Q : Inport  Port=2
  Add : Sum
  Divide : Product  Inputs=*/
  Product : Product
  Product1 : Product
  Square Root : Sqrt  SaturateOnIntegerOverflow=on
  Out1 : Outport
  wires:
  Divide/1 -> Out1/1
  P/1 -> Divide/1, Product/2, Product/1
  Product/1 -> Add/1
  Add/1 -> Square Root/1
  Q/1 -> Product1/1, Product1/2
  Square Root/1 -> Divide/2
  Product1/1 -> Add/2

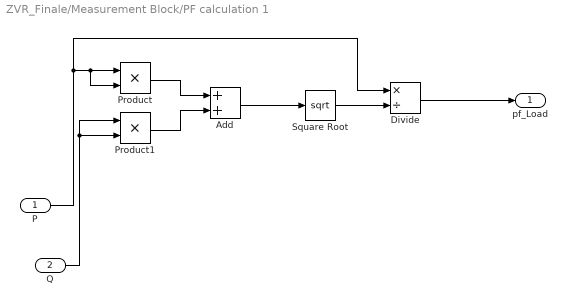
== system ZVR_Finale/Measurement Block/PF calculation 1 ==
  P : Inport
  Q : Inport  Port=2
  Add : Sum
  Divide : Product  Inputs=*/
  Product : Product
  Product1 : Product
  Square Root : Sqrt  SaturateOnIntegerOverflow=on
  pf_Load : Outport
  wires:
  Divide/1 -> pf_Load/1
  P/1 -> Divide/1, Product/2, Product/1
  Product/1 -> Add/1
  Add/1 -> Square Root/1
  Q/1 -> Product1/1, Product1/2
  Square Root/1 -> Divide/2
  Product1/1 -> Add/2

== system ZVR_Finale/Measurement Block/PF calculation 2 ==
  P : Inport
  Q : Inport  Port=2
  Add : Sum
  Divide : Product  Inputs=*/
  Product : Product
  Product1 : Product
  Square Root : Sqrt  SaturateOnIntegerOverflow=on
  Out1 : Outport
  wires:
  Divide/1 -> Out1/1
  P/1 -> Divide/1, Product/2, Product/1
  Product/1 -> Add/1
  Add/1 -> Square Root/1
  Q/1 -> Product1/1, Product1/2
  Square Root/1 -> Divide/2
  Product1/1 -> Add/2

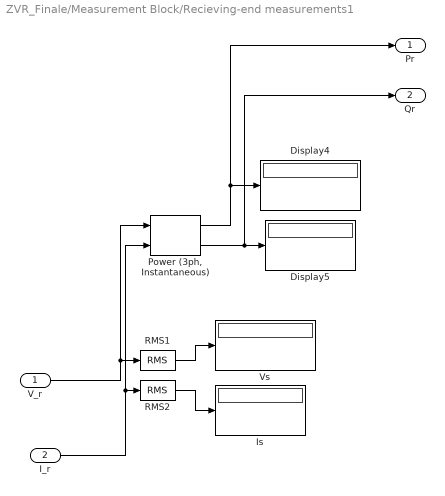
== system ZVR_Finale/Measurement Block/Recieving-end measurements1 ==
  V_r : Inport
  I_r : Inport  Port=2
  Display4 : Display
  Display5 : Display
  Is : Display
  "Power (3ph, Instantaneous)" : powerlib_meascontrol/Measurements/Power (3ph, Instantaneous)
      settings: SourceProductName=Simscape Electrical
  RMS1 : powerlib_meascontrol/Measurements/RMS  TrueRMS=on  Freq=60  RMSInit=120  Ts=0
      settings: SourceProductName=Simscape Electrical
  RMS2 : powerlib_meascontrol/Measurements/RMS  TrueRMS=on  Freq=60  RMSInit=120  Ts=0
      settings: SourceProductName=Simscape Electrical
  Vs : Display
  Pr : Outport
  Qr : Outport  Port=2
  wires:
  RMS2/1 -> Is/1
  "Power (3ph, Instantaneous)"/1 -> Pr/1, Display4/1
  "Power (3ph, Instantaneous)"/2 -> Qr/1, Display5/1
  V_r/1 -> "Power (3ph, Instantaneous)"/1, RMS1/1
  I_r/1 -> "Power (3ph, Instantaneous)"/2, RMS2/1
  RMS1/1 -> Vs/1

== system ZVR_Finale/Measurement Block/Sending-end measurements ==
  V_s : Inport
  I_s : Inport  Port=2
  "Power (3ph, Instantaneous)" : powerlib_meascontrol/Measurements/Power (3ph, Instantaneous)
      settings: SourceProductName=Simscape Electrical
  Ps : Outport
  Qs : Outport  Port=2
  wires:
  "Power (3ph, Instantaneous)"/1 -> Ps/1
  "Power (3ph, Instantaneous)"/2 -> Qs/1
  V_s/1 -> "Power (3ph, Instantaneous)"/1
  I_s/1 -> "Power (3ph, Instantaneous)"/2

== system ZVR_Finale/Measurement Block/Sending-end measurements2 ==
  V_s : Inport
  I_s : Inport  Port=2
  "Power (3ph, Instantaneous)" : powerlib_meascontrol/Measurements/Power (3ph, Instantaneous)
      settings: SourceProductName=Simscape Electrical
  Ps : Outport
  Qs : Outport  Port=2
  wires:
  "Power (3ph, Instantaneous)"/1 -> Ps/1
  "Power (3ph, Instantaneous)"/2 -> Qs/1
  V_s/1 -> "Power (3ph, Instantaneous)"/1
  I_s/1 -> "Power (3ph, Instantaneous)"/2

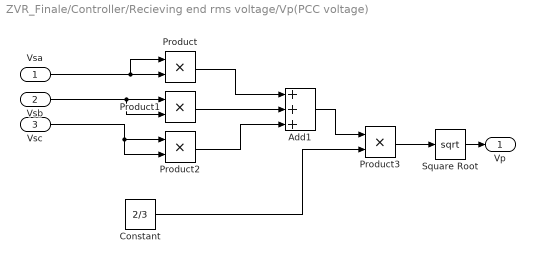
== system ZVR_Finale/Controller/Recieving end rms voltage/Vp(PCC voltage) ==
  Vsa : Inport
  Vsb : Inport  Port=2
  Vsc : Inport  Port=3
  Add1 : Sum  Inputs=+++
  Constant : Constant  Value=2/3
  Product{,1..3} (4 alike) : Product
  Square Root : Sqrt  SaturateOnIntegerOverflow=on
  Vp : Outport
  wires:
  Vsc/1 -> Product2/2, Product2/1
  Product1/1 -> Add1/2
  Add1/1 -> Product3/1
  Vsa/1 -> Product/1, Product/2
  Vsb/1 -> Product1/2, Product1/1
  Product3/1 -> Square Root/1
  Square Root/1 -> Vp/1
  Product2/1 -> Add1/3
  Product/1 -> Add1/1
  Constant/1 -> Product3/2

== matlab function ZVR_Finale/Controller/IN-Phase-components ==
  data: idls input; vsa input; isa_star output; vsb input; vsc input; isb_star output; isc_star output; usa output; usb output; usc output; vp output
function [isa_star , isb_star ,isc_star,usa,usb,usc,vp] = fcn(idls,vsa,vsb,vsc)

vp = sqrt((2/3)*(vsa^2+vsb^2+vsc^2));

usa = vsa/vp;

usb = vsb / vp;

usc = vsc /vp;

isa_star = usa*idls;

isb_star = usb * idls;

isc_star = usc*idls;
